simulink model "RmtAPP_Kickdown"  (R2016b)
settings: configuration reference "CodeGenConfigSet" (kept outside this file)
values from neighbouring files (symbols this model uses):
  MoFRmtAPP_dRawSigFac_C = Calibration.Parameter    [init_RmtAPP_Kickdown.m]    (also in init_RmtAPP_Kickdown_SIL.m = Simulink.Parameter)
  RmtAPP_stAPPChannelNum_C = Calibration.Parameter    [init_RmtAPP_Kickdown.m]    (also in init_RmtAPP_Kickdown_SIL.m = Simulink.Parameter)
  RmtAPP_uKDHighAPP_C = Calibration.Parameter    [init_RmtAPP_Kickdown.m]    (also in init_RmtAPP_Kickdown_SIL.m = Simulink.Parameter)
  RmtAPP_uKDLowAPP_C = Calibration.Parameter    [init_RmtAPP_Kickdown.m]    (also in init_RmtAPP_Kickdown_SIL.m = Simulink.Parameter)
  SigTst_stRmtAPPKickDown_C = Calibration.Parameter    [init_RmtAPP_Kickdown.m]    (also in init_RmtAPP_Kickdown_SIL.m = Simulink.Parameter)
  SigTst_swtRmtAPPKickDown_C = Calibration.Parameter    [init_RmtAPP_Kickdown.m]    (also in init_RmtAPP_Kickdown_SIL.m = Simulink.Parameter)
undefined symbols (not defined in the file or in its folder): Switch_conv
libraries: CXLib x2
settings Model: Creator=bianxuyin  LastModifiedBy=xuxingpei
settings ConfigSetRef: SourceLocation=Base Workspace

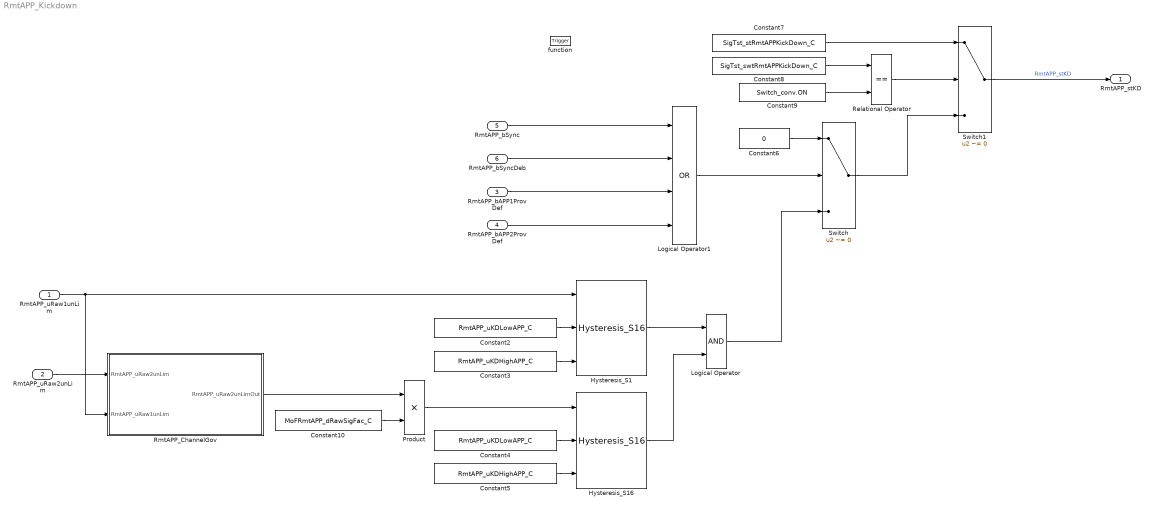
== system RmtAPP_Kickdown ==
  RmtAPP_uRaw1unLim : Inport  Tag=mv  Description=Remote Acceleration pedal sensor 1 unlimited raw value  OutMin=0  OutMax=5000  OutDataTypeStr=Ad_mv
  RmtAPP_uRaw2unLim : Inport  Tag=mv  Description=Remote Acceleration pedal sensor 2 unlimited raw value  Port=2  OutMin=0  OutMax=5000  OutDataTypeStr=Ad_mv
  RmtAPP_bAPP1ProvDef : Inport  Description=Status Sensor 1 of the remote acceleration pedal temporary defect  Port=3  OutMin=0  OutMax=1  OutDataTypeStr=boolean
  RmtAPP_bAPP2ProvDef : Inport  Description=Status Sensor 2 of the remote acceleration pedal temporary defect  Port=4  OutMin=0  OutMax=1  OutDataTypeStr=boolean
  RmtAPP_bSync : Inport  Description=Status temporary sync check  Port=5  OutMin=0  OutMax=1  OutDataTypeStr=boolean
  RmtAPP_bSyncDeb : Inport  Description=Status debounced sync check  Port=6  OutMin=0  OutMax=1  OutDataTypeStr=boolean
  function : TriggerPort  TriggerType=function-call  VariantControl=Variant
  Constant10 : Constant  Value=MoFRmtAPP_dRawSigFac_C  SampleTime=-1
  Constant2 : Constant  Value=RmtAPP_uKDLowAPP_C
  Constant3 : Constant  Value=RmtAPP_uKDHighAPP_C
  Constant4 : Constant  Value=RmtAPP_uKDLowAPP_C
  Constant5 : Constant  Value=RmtAPP_uKDHighAPP_C
  Constant6 : Constant  Value=0  OutDataTypeStr=Inherit: Inherit via back propagation
  Constant7 : Constant  Value=SigTst_stRmtAPPKickDown_C
  Constant8 : Constant  Value=SigTst_swtRmtAPPKickDown_C
  Constant9 : Constant  Value=Switch_conv.ON  OutDataTypeStr=Inherit: Inherit via back propagation
  Hysteresis_S1 : CXLib/Hysteresis_S16
  Hysteresis_S16 : CXLib/Hysteresis_S16
  Logical Operator : Logic  AllPortsSameDT=off  OutDataTypeStr=boolean
  Logical Operator1 : Logic  Operator=OR  Inputs=4  AllPortsSameDT=off  OutDataTypeStr=boolean
  Product : Product  OutDataTypeStr=Ad_mv
  Relational Operator : RelationalOperator  Operator===  OutDataTypeStr=boolean  RndMeth=Simplest
  RmtAPP_ChannelGov : Subsystem
  Switch : Switch  Criteria=u2 ~= 0
  Switch1 : Switch  Criteria=u2 ~= 0
  RmtAPP_stKD : Outport  Description="State of  remot accelerator pedal kick down"  OutMin=0  OutMax=1  OutDataTypeStr=boolean
  wires:
  Switch1/1 -> RmtAPP_stKD/1  "RmtAPP_stKD"
  RmtAPP_uRaw1unLim/1 -> RmtAPP_ChannelGov/2(RmtAPP_uRaw1unLim), Hysteresis_S1/1
  Constant2/1 -> Hysteresis_S1/2
  Constant3/1 -> Hysteresis_S1/3
  Constant10/1 -> Product/2
  Product/1 -> Hysteresis_S16/1
  Constant4/1 -> Hysteresis_S16/2
  Constant5/1 -> Hysteresis_S16/3
  Hysteresis_S1/1 -> Logical Operator/1
  Hysteresis_S16/1 -> Logical Operator/2
  Logical Operator/1 -> Switch/3
  Logical Operator1/1 -> Switch/2
  RmtAPP_bSync/1 -> Logical Operator1/1
  RmtAPP_bSyncDeb/1 -> Logical Operator1/2
  RmtAPP_bAPP1ProvDef/1 -> Logical Operator1/3
  RmtAPP_bAPP2ProvDef/1 -> Logical Operator1/4
  Constant6/1 -> Switch/1
  Switch/1 -> Switch1/3
  Relational Operator/1 -> Switch1/2
  Constant9/1 -> Relational Operator/2
  Constant8/1 -> Relational Operator/1
  Constant7/1 -> Switch1/1
  RmtAPP_uRaw2unLim/1 -> RmtAPP_ChannelGov/1(RmtAPP_uRaw2unLim)
  RmtAPP_ChannelGov/1(RmtAPP_uRaw2unLimOut) -> Product/1

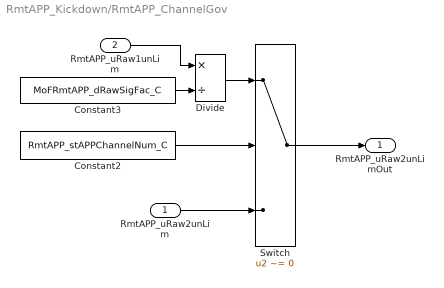
== system RmtAPP_Kickdown/RmtAPP_ChannelGov ==
  RmtAPP_uRaw2unLim : Inport  Tag=mv  Description=Remote Acceleration pedal sensor 2 unlimited raw value  OutMin=0  OutMax=5000  OutDataTypeStr=Ad_mv
  RmtAPP_uRaw1unLim : Inport  Tag=mv  Description=Remote Acceleration pedal sensor 1 unlimited raw value  Port=2  OutMin=0  OutMax=5000  OutDataTypeStr=Ad_mv
  Constant2 : Constant  Value=RmtAPP_stAPPChannelNum_C
  Constant3 : Constant  Value=MoFRmtAPP_dRawSigFac_C  SampleTime=-1
  Divide : Product  Inputs=*/  OutDataTypeStr=Inherit: Inherit via back propagation  SaturateOnIntegerOverflow=on
  Switch : Switch  Criteria=u2 ~= 0
  RmtAPP_uRaw2unLimOut : Outport
  wires:
  RmtAPP_uRaw1unLim/1 -> Divide/1
  Constant2/1 -> Switch/2
  Switch/1 -> RmtAPP_uRaw2unLimOut/1
  Constant3/1 -> Divide/2
  RmtAPP_uRaw2unLim/1 -> Switch/3
  Divide/1 -> Switch/1
